simulink model "Sim6_03_lim_current_LCL"  (R2019b)
settings: Solver=ode1  StartTime=0.0  StopTime=1.5  FixedStep=Time_Step  MaxStep=1e-5  RelTol=1e-3
undefined symbols (not defined in the file): C_line, L_1, L_2, R_1, R_2, Theta0, Time_Step, Un, V0, VSC01_id0
libraries: powerlib x37, Control_Lib x7, simulink x5, powerlib_meascontrol x4
(part 2 of 2)

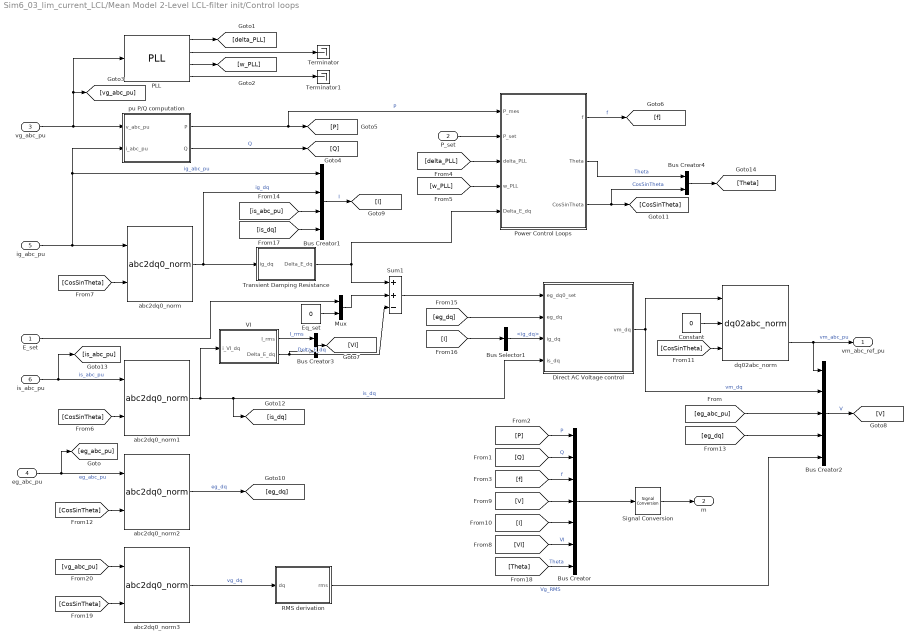
== system Sim6_03_lim_current_LCL/Mean Model 2-Level LCL-filter init/Control loops ==
  E_set : Inport
  P_set : Inport  Port=2
  vg_abc_pu : Inport  Port=3
  eg_abc_pu : Inport  Port=4
  ig_abc_pu : Inport  Port=5
  is_abc_pu : Inport  Port=6
  " pu P/Q computation" : Subsystem  DialogController=POWERSYS.PowerSysDialog
  Bus Creator : BusCreator  Inputs=7
  Bus Creator1 : BusCreator  Inputs=4
  Bus Creator2 : BusCreator  Inputs=5
  Bus Creator3 : BusCreator  Inputs=2
  Bus Creator4 : BusCreator  Inputs=2
  Bus Selector1 : BusSelector  OutputSignals=ig_dq
  Constant : Constant  Value=0
  Direct AC Voltage control : Subsystem
  Eq_set : Constant  Value=0
  Mux : Mux  Inputs=2
  PLL : Control_Lib/PLL  fb=fb  Tr_PLL=Tr_PLL  Theta0=Theta0
      settings: SourceProductName=VSC4SPS
  Power Control Loops : Subsystem
  RMS derivation : Subsystem
  Signal Conversion : SignalConversion  OverrideOpt=off
  Sum1 : Sum  Inputs=++-
  Terminator : Terminator
  Terminator1 : Terminator
  Transient Damping Resistance : Subsystem
  VI : Subsystem
  abc2dq0_norm{,1..3} (4 alike) : Control_Lib/abc2dq0_norm  referenceAxisMode=Reference axis at 90 degrees behind phase_a  baseUpdateGain=1/sqrt(3)
      settings: SourceProductName=VSC4SPS
  dq02abc_norm : Control_Lib/dq02abc_norm  referenceAxisMode=Reference axis at 90 degrees behind phase_a  baseUpdateGain=sqrt(3)
      settings: SourceProductName=VSC4SPS
  vm_abc_ref_pu : Outport  PortDimensions=3  VectorParamsAs1DForOutWhenUnconnected=off
  m : Outport  Port=2  VectorParamsAs1DForOutWhenUnconnected=off
  wires:
  [w_PLL] -> Power Control Loops/4(w_PLL)
  RMS derivation/1(rms) -> Bus Creator2/5  "Vg_RMS"
  abc2dq0_norm3/2 -> RMS derivation/1(dq)  "vg_dq"
  [vg_abc_pu] -> abc2dq0_norm3/1
  [CosSinTheta] -> abc2dq0_norm3/2
  [Theta] -> Bus Creator/7  "Theta"
  Bus Creator4/1 -> [Theta]
  Power Control Loops/2(Theta) -> Bus Creator4/1  "Theta"
  Power Control Loops/3(CosSinTheta) -> [CosSinTheta], Bus Creator4/2  "CosSinTheta"
  PLL/4 -> Terminator1/1
  PLL/2 -> Terminator/1
  Constant/1 -> dq02abc_norm/2
  PLL/3 -> [w_PLL]
  PLL/1 -> [delta_PLL]
  Sum1/1 -> Direct AC Voltage control/1(eg_dq0_set)
  [I] -> Bus Selector1/1
  Bus Selector1/1 -> Direct AC Voltage control/3(ig_dq)  "<ig_dq>"
  Bus Creator2/1 -> [V]  "V"
  [CosSinTheta] -> dq02abc_norm/3
  dq02abc_norm/2 -> vm_abc_ref_pu/1, Bus Creator2/1  "vm_abc_pu"
  Direct AC Voltage control/1(vm_dq) -> Bus Creator2/2, dq02abc_norm/1  "vm_dq"
  [eg_dq] -> Direct AC Voltage control/2(eg_dq)
  eg_abc_pu/1 -> [eg_abc_pu], abc2dq0_norm2/1  "eg_abc_pu"
  is_abc_pu/1 -> abc2dq0_norm1/1, [is_abc_pu]  "is_abc_pu"
  abc2dq0_norm2/2 -> [eg_dq]  "eg_dq"
  [CosSinTheta] -> abc2dq0_norm2/2
  abc2dq0_norm1/2 -> [is_dq], Direct AC Voltage control/4(is_dq), VI/1(i_VI_dq)  "is_dq"
  vg_abc_pu/1 -> PLL/1, [vg_abc_pu], " pu P/Q computation"/1(v_abc_pu)
  [CosSinTheta] -> abc2dq0_norm1/2
  [I] -> Bus Creator/5
  Bus Creator1/1 -> [I]  "I"
  Bus Creator/1 -> Signal Conversion/1
  [VI] -> Bus Creator/6  "VI"
  [V] -> Bus Creator/4
  Eq_set/1 -> Mux/2
  Mux/1 -> Sum1/2
  VI/1(I_rms) -> Bus Creator3/1  "I_rms"
  Transient Damping Resistance/1("Delta_E_dq ") -> Sum1/1, Power Control Loops/5(Delta_E_dq)
  VI/2(Delta_E_dq) -> Sum1/3, Bus Creator3/2  "Delta_E_dq"
  [CosSinTheta] -> abc2dq0_norm/2
  abc2dq0_norm/2 -> Transient Damping Resistance/1(ig_dq), Bus Creator1/2  "ig_dq"
  ig_abc_pu/1 -> " pu P/Q computation"/2(i_abc_pu), Bus Creator1/1, abc2dq0_norm/1  "ig_abc_pu"
  " pu P/Q computation"/1(P) -> [P], Power Control Loops/1(P_mes)  "P"
  Power Control Loops/1(f) -> [f]  "f"
  P_set/1 -> Power Control Loops/2(P_set)
  [delta_PLL] -> Power Control Loops/3(delta_PLL)
  " pu P/Q computation"/2(Q) -> [Q]  "Q"
  E_set/1 -> Mux/1
  [f] -> Bus Creator/3  "f"
  [Q] -> Bus Creator/2  "Q"
  [P] -> Bus Creator/1  "P"
  Signal Conversion/1 -> m/1
  Bus Creator3/1 -> [VI]
  [eg_abc_pu] -> Bus Creator2/3
  [eg_dq] -> Bus Creator2/4
  [is_abc_pu] -> Bus Creator1/3
  [is_dq] -> Bus Creator1/4

== system Sim6_03_lim_current_LCL/Mean Model 2-Level LCL-filter init/Output_Filter ==
  Filter capacitance : powerlib/Elements/Three-Phase Series RLC Branch  LConnTagsString=A|B|C  RConnTagsString=A|B|C  BranchType=C  Resistance=0  Inductance=C_line(1)  Capacitance=Cf_pu*Cb  Measurements=None
  Filter inductance : powerlib/Elements/Three-Phase Series RLC Branch  LConnTagsString=A|B|C  RConnTagsString=A|B|C  BranchType=RL  Resistance=Rf_pu*Zb  Inductance=Lf_pu*Lb  Capacitance=1e-6  Measurements=None
  Ground : powerlib/Elements/Ground  LConnTagsString=a
  A : PMIOPort  Side=Left
  a : PMIOPort  Port=2  Side=Right
  B : PMIOPort  Port=3  Side=Left
  b : PMIOPort  Port=4  Side=Right
  C : PMIOPort  Port=5  Side=Left
  c : PMIOPort  Port=6  Side=Right
  connections:
  Ground/LConn1 -- Filter capacitance/RConn1 -- Filter capacitance/RConn3 -- Filter capacitance/RConn2
  b/RConn1 -- Filter capacitance/LConn2 -- Filter inductance/RConn2
  Filter inductance/LConn1 -- A/RConn1
  Filter inductance/LConn3 -- C/RConn1
  Filter inductance/LConn2 -- B/RConn1
  c/RConn1 -- Filter capacitance/LConn3 -- Filter inductance/RConn3
  a/RConn1 -- Filter capacitance/LConn1 -- Filter inductance/RConn1

== system Sim6_03_lim_current_LCL/Infinite_Grid/InertialDqVoltageSource/NetworkLeadLagTimeConstants ==
  In1 : Inport
  Integrator3 : Integrator  InitialCondition=(P0/Sb)*(1-TN/TD)
  Sum1 : Sum
  Sum2 : Sum  Inputs=+-
  mp1 : Gain  Gain=TN/TD
  mp2 : Gain  Gain=1-TN/TD
  mp3 : Gain  Gain=1/TD
  Out1 : Outport  VectorParamsAs1DForOutWhenUnconnected=off
  wires:
  Sum2/1 -> mp3/1
  mp3/1 -> Integrator3/1
  Integrator3/1 -> Sum1/2, Sum2/2
  In1/1 -> mp1/1, mp2/1
  mp2/1 -> Sum2/1
  mp1/1 -> Sum1/1
  Sum1/1 -> Out1/1

== system Sim6_03_lim_current_LCL/Infinite_Grid/Source_For_OP/Subsystem3 ==
  switch : Inport
  Breaker : powerlib/Elements/Breaker  InitialState=0  SwitchingTimes="[1/60  5/60]"  External=on  BreakerResistance=0.001  SnubberResistance=1e6  SnubberCapacitance=inf  Measurements=None  MoreParameters=on  NoBreakLoop=off
  Breaker1 : powerlib/Elements/Breaker  InitialState=0  SwitchingTimes="[1/60  5/60]"  External=on  BreakerResistance=0.001  SnubberResistance=1e6  SnubberCapacitance=inf  Measurements=None  MoreParameters=on  NoBreakLoop=off
  Breaker2 : powerlib/Elements/Breaker  InitialState=0  SwitchingTimes="[1/60  5/60]"  External=on  BreakerResistance=0.001  SnubberResistance=1e6  SnubberCapacitance=inf  Measurements=None  MoreParameters=on  NoBreakLoop=off
  Breaker3 : powerlib/Elements/Breaker  InitialState=1  SwitchingTimes="[1/60  5/60]"  External=on  BreakerResistance=0.001  SnubberResistance=1e6  SnubberCapacitance=inf  Measurements=None  MoreParameters=on  NoBreakLoop=off
  Breaker4 : powerlib/Elements/Breaker  InitialState=1  SwitchingTimes="[1/60  5/60]"  External=on  BreakerResistance=0.001  SnubberResistance=1e6  SnubberCapacitance=inf  Measurements=None  MoreParameters=on  NoBreakLoop=off
  Breaker5 : powerlib/Elements/Breaker  InitialState=1  SwitchingTimes="[1/60  5/60]"  External=on  BreakerResistance=0.001  SnubberResistance=1e6  SnubberCapacitance=inf  Measurements=None  MoreParameters=on  NoBreakLoop=off
  Logical Operator : Logic  Operator=NOT  AllPortsSameDT=off  OutDataTypeStr=boolean
  A : PMIOPort  Side=Left
  B : PMIOPort  Port=2  Side=Left
  C : PMIOPort  Port=3  Side=Left
  Ainit : PMIOPort  Port=4  Side=Left
  Binit : PMIOPort  Port=5  Side=Left
  Cinit : PMIOPort  Port=6  Side=Left
  a : PMIOPort  Port=7  Side=Right
  b : PMIOPort  Port=8  Side=Right
  c : PMIOPort  Port=9  Side=Right
  wires:
  Logical Operator/1 -> Breaker3/1, Breaker4/1, Breaker5/1
  switch/1 -> Logical Operator/1, Breaker/1, Breaker1/1, Breaker2/1
  connections:
  Breaker4/RConn1 -- Breaker1/RConn1 -- b/RConn1
  a/RConn1 -- Breaker3/RConn1 -- Breaker/RConn1
  Breaker1/LConn1 -- B/RConn1
  Breaker3/LConn1 -- Ainit/RConn1
  Breaker2/LConn1 -- C/RConn1
  Breaker4/LConn1 -- Binit/RConn1
  Breaker2/RConn1 -- Breaker5/RConn1 -- c/RConn1
  Breaker5/LConn1 -- Cinit/RConn1
  Breaker/LConn1 -- A/RConn1

== system Sim6_03_lim_current_LCL/Mean Model 2-Level LCL-filter init/Bridge_Model/Detailed ==
  Urref : Inport
  Bus Selector : BusSelector  OutputSignals=carrier
  PWM Generator (2-Level) : powerlib_meascontrol/Pulse & Signal Generators/PWM Generator (2-Level)  ModulatorType=Three-phase bridge (6 pulses)  ModulatorMode=Unsynchronized  Fc=fpwm  Pc=90  nF=27  MinMax="[ -1  1 ]"  SamplingTechnique=Natural  ModulatingSignals=off  m=0.8  Freq=60  Phase=0  Ts=Time_Step  ShowCarrierOutport=on
  Scope : Scope
  Scope1 : Scope
  Universal Bridge1 : powerlib/Power Electronics/Universal Bridge  Arms=3  SnubberResistance=1e5  SnubberCapacitance=inf  Device=IGBT / Diodes  Ron=1e-3  Lon=0  ForwardVoltages="[  0  0  ]"  ForwardVoltage=0  GTOparameters=[ 10e-6 , 20e-6 ]  IGBTparameters=[ 1e-6 , 2e-6 ]  Measurements=None  Measurements_2=None  converterType=Rectifier
  + : PMIOPort  Side=Right
  A : PMIOPort  Port=2  Side=Left
  B : PMIOPort  Port=3  Side=Left
  - : PMIOPort  Port=4  Side=Right
  C : PMIOPort  Port=5  Side=Left
  wires:
  PWM Generator (2-Level)/1 -> Universal Bridge1/1, Scope1/1
  Urref/1 -> PWM Generator (2-Level)/1
  PWM Generator (2-Level)/2 -> Bus Selector/1
  Bus Selector/1 -> Scope/1  "<carrier>"
  connections:
  Universal Bridge1/LConn3 -- C/RConn1
  Universal Bridge1/LConn1 -- A/RConn1
  Universal Bridge1/LConn2 -- B/RConn1
  Universal Bridge1/RConn2 -- -/RConn1
  Universal Bridge1/RConn1 -- +/RConn1

== system Sim6_03_lim_current_LCL/Mean Model 2-Level LCL-filter init/Control loops/ pu P//Q computation ==
  v_abc_pu : Inport  PortDimensions=3
  i_abc_pu : Inport  Port=2  PortDimensions=3
  Demux : Demux  Outputs=3
      settings: DisplayOption=none
  Mux : Mux  Inputs=3
  Product1 : Product  InputSameDT=on  SaturateOnIntegerOverflow=on  OutDataTypeStr=Inherit: Same as first input
  Product3 : Product  InputSameDT=on  SaturateOnIntegerOverflow=on  OutDataTypeStr=Inherit: Same as first input
  Sum : Sum  Inputs=+-  InputSameDT=on  SaturateOnIntegerOverflow=on  OutDataTypeStr=Inherit: Same as first input
  Sum1 : Sum  Inputs=1  InputSameDT=on  SaturateOnIntegerOverflow=on  OutDataTypeStr=Inherit: Same as first input
  Sum4 : Sum  Inputs=1  InputSameDT=on  SaturateOnIntegerOverflow=on  OutDataTypeStr=Inherit: Same as first input
  Sum5 : Sum  Inputs=+-  InputSameDT=on  SaturateOnIntegerOverflow=on  OutDataTypeStr=Inherit: Same as first input
  Sum6 : Sum  Inputs=+-  InputSameDT=on  SaturateOnIntegerOverflow=on  OutDataTypeStr=Inherit: Same as first input
  pu->V : Gain  Gain=1/sqrt(3)  SaturateOnIntegerOverflow=on  OutDataTypeStr=Inherit: Same as input  ParamDataTypeStr=Inherit: Same as input
  pu->V1 : Gain  Gain=1/3  SaturateOnIntegerOverflow=on  OutDataTypeStr=Inherit: Same as input  ParamDataTypeStr=Inherit: Same as input
  pu->V2 : Gain  Gain=1/3  SaturateOnIntegerOverflow=on  OutDataTypeStr=Inherit: Same as input  ParamDataTypeStr=Inherit: Same as input
  P : Outport  VectorParamsAs1DForOutWhenUnconnected=off
  Q : Outport  Port=2  VectorParamsAs1DForOutWhenUnconnected=off
  wires:
  pu->V2/1 -> Q/1
  pu->V1/1 -> P/1
  Sum1/1 -> pu->V/1
  Product3/1 -> Sum1/1
  Product1/1 -> Sum4/1
  v_abc_pu/1 -> Product1/1, Demux/1
  i_abc_pu/1 -> Product1/2, Product3/2
  Sum4/1 -> pu->V1/1
  Demux/1 -> Sum/1, Sum6/2
  Demux/2 -> Sum/2, Sum5/1
  Demux/3 -> Sum5/2, Sum6/1
  Sum/1 -> Mux/3
  Sum5/1 -> Mux/1
  Sum6/1 -> Mux/2
  Mux/1 -> Product3/1
  pu->V/1 -> pu->V2/1  "Q"

== system Sim6_03_lim_current_LCL/Mean Model 2-Level LCL-filter init/Control loops/Direct AC Voltage control ==
  note: direct AC voltage control
  eg_dq0_set : Inport
  eg_dq : Inport  Port=2
  ig_dq : Inport  Port=3
  is_dq : Inport  Port=4
  Current Limitation : Subsystem
  Gain : Gain  Gain=RLCL_D
  Gain2 : Gain  Gain=[Rf_pu -Lf_pu;Lf_pu Rf_pu]  Multiplication=Matrix(K*u)
  Second-Order Filter : powerlib_meascontrol/Filters/Second-Order Filter  FilterType=Highpass  Fo=f_damping  Zeta=1  Ts=0  Initialize=on  Vac_Init="[0,  0,  60; 0, 0, 60]"  Vdc_Init=[0, 0]  PlotResponse=off  FreqRange=[0, 500, 1]
      settings: SourceProductBaseCode=PS
  Second-Order Filter1 : powerlib_meascontrol/Filters/Second-Order Filter  FilterType=Lowpass  Fo=f_damping  Zeta=1  Ts=0  Initialize=on  Vac_Init="[0,  0,  60; 0 0 60]"  Vdc_Init=[Is0_d; Is0_q]  PlotResponse=off  FreqRange=[0, 500, 1]
      settings: SourceProductBaseCode=PS
  Second-Order Filter2 : powerlib_meascontrol/Filters/Second-Order Filter  FilterType=Lowpass  Fo=1000  Zeta=1  Ts=0  Initialize=on  Vac_Init="[0,  0,  60; 0, 0, 60]"  Vdc_Init=[0, 0]  PlotResponse=off  FreqRange=[0, 500, 1]
      settings: SourceProductBaseCode=PS
  Sum : Sum  Inputs=|++
  Sum1 : Sum  Inputs=|+-
  Sum2 : Sum  Inputs=-+|
  vm_dq : Outport  VectorParamsAs1DForOutWhenUnconnected=off
  wires:
  ig_dq/1 -> Sum1/2
  eg_dq/1 -> Current Limitation/3(Eg_dq)
  is_dq/1 -> Second-Order Filter1/1, Current Limitation/2(Is_dq), Sum1/1
  eg_dq0_set/1 -> Sum/2
  Sum/1 -> Sum2/2
  Sum1/1 -> Second-Order Filter/1
  Second-Order Filter/1 -> Second-Order Filter2/1
  Gain/1 -> Sum2/1
  Sum2/1 -> Current Limitation/1(Vm_dq*)
  Gain2/1 -> Sum/1
  Second-Order Filter1/1 -> Gain2/1
  Second-Order Filter2/1 -> Gain/1
  Current Limitation/1(Vm_dq_sat) -> vm_dq/1

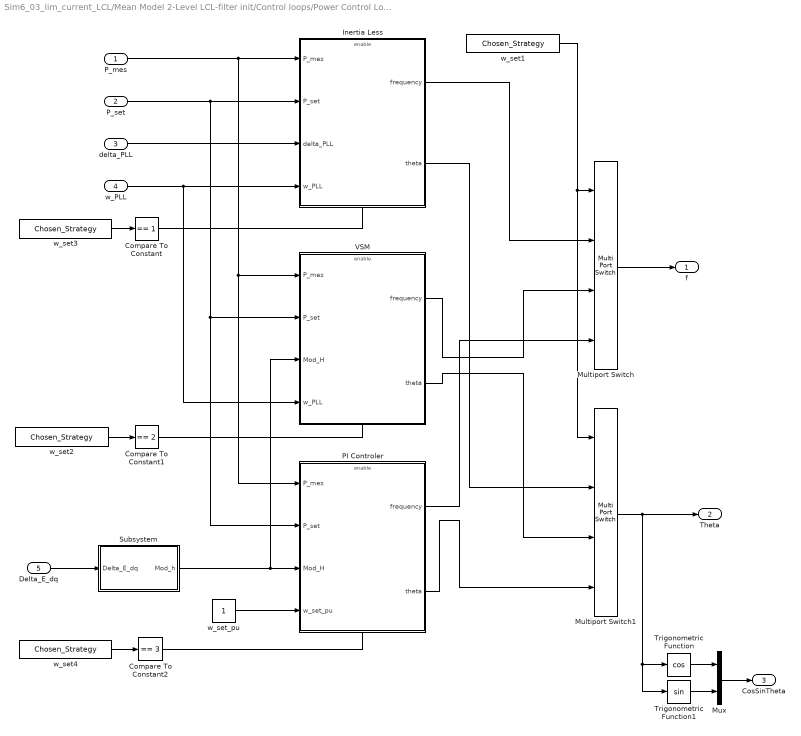
== system Sim6_03_lim_current_LCL/Mean Model 2-Level LCL-filter init/Control loops/Power Control Loops ==
  P_mes : Inport
  P_set : Inport  Port=2
  delta_PLL : Inport  Port=3
  w_PLL : Inport  Port=4
  Delta_E_dq : Inport  Port=5
  Compare To Constant : simulink/Logic and Bit Operations/Compare To Constant  relop===  const=1  OutDataTypeStr=boolean
  Compare To Constant1 : simulink/Logic and Bit Operations/Compare To Constant  relop===  const=2  OutDataTypeStr=boolean
  Compare To Constant2 : simulink/Logic and Bit Operations/Compare To Constant  relop===  const=3  OutDataTypeStr=boolean
  Inertia Less : Subsystem
  Multiport Switch : MultiPortSwitch
  Multiport Switch1 : MultiPortSwitch
  Mux : Mux  Inputs=[1 1]
  PI Controler : Subsystem
  Subsystem : Subsystem
  Trigonometric Function : Trigonometry  Operator=cos
  Trigonometric Function1 : Trigonometry
  VSM : Subsystem
  w_set{1..4} (4 alike) : Constant  Value=Chosen_Strategy
  w_set_pu : Constant
  f : Outport  PortDimensions=1  VectorParamsAs1DForOutWhenUnconnected=off
  Theta : Outport  Port=2  VectorParamsAs1DForOutWhenUnconnected=off
  CosSinTheta : Outport  Port=3  PortDimensions=2  VectorParamsAs1DForOutWhenUnconnected=off
  wires:
  P_mes/1 -> PI Controler/1(P_mes), VSM/1(P_mes), Inertia Less/1(P_mes)
  P_set/1 -> PI Controler/2(P_set), VSM/2(P_set), Inertia Less/2(P_set)
  delta_PLL/1 -> Inertia Less/3(delta_PLL)
  w_PLL/1 -> VSM/4(w_PLL), Inertia Less/4(w_PLL)
  w_set_pu/1 -> PI Controler/4(w_set_pu)
  PI Controler/2(theta) -> Multiport Switch1/4
  PI Controler/1(frequency) -> Multiport Switch/4
  VSM/1(frequency) -> Multiport Switch/3
  w_set1/1 -> Multiport Switch1/1, Multiport Switch/1
  VSM/2(theta) -> Multiport Switch1/3
  Inertia Less/2(theta) -> Multiport Switch1/2
  Multiport Switch/1 -> f/1
  Inertia Less/1(frequency) -> Multiport Switch/2
  w_set3/1 -> Compare To Constant/1
  w_set2/1 -> Compare To Constant1/1
  w_set4/1 -> Compare To Constant2/1
  Compare To Constant/1 -> Inertia Less/Enable
  Compare To Constant1/1 -> VSM/Enable
  Compare To Constant2/1 -> PI Controler/Enable
  Trigonometric Function/1 -> Mux/1
  Mux/1 -> CosSinTheta/1
  Trigonometric Function1/1 -> Mux/2
  Multiport Switch1/1 -> Theta/1, Trigonometric Function/1, Trigonometric Function1/1
  Delta_E_dq/1 -> Subsystem/1(Delta_E_dq)
  Subsystem/1(Mod_h) -> VSM/3(Mod_H), PI Controler/3(Mod_H)

== system Sim6_03_lim_current_LCL/Mean Model 2-Level LCL-filter init/Control loops/RMS derivation ==
  dq : Inport
  Demux : Demux  Outputs=2
  Sqrt : Sqrt  SaturateOnIntegerOverflow=on
  Square : Math  Operator=square  SaturateOnIntegerOverflow=on
  Square1 : Math  Operator=square  SaturateOnIntegerOverflow=on
  Sum : Sum
  rms : Outport
  wires:
  Square1/1 -> Sum/2
  Sum/1 -> Sqrt/1
  Sqrt/1 -> rms/1
  Demux/1 -> Square/1
  Square/1 -> Sum/1
  Demux/2 -> Square1/1
  dq/1 -> Demux/1

== system Sim6_03_lim_current_LCL/Mean Model 2-Level LCL-filter init/Control loops/Transient Damping Resistance ==
  ig_dq : Inport
  Filter w_LF : Subsystem
      mask Display: disp('\omega_{LF} / (s + \omega_{LF})','texmode','on')
  Sum5 : Sum  Inputs=|+-
  nq1 : Gain  Gain=Rv
  "Delta_E_dq " : Outport  VectorParamsAs1DForOutWhenUnconnected=off
  wires:
  nq1/1 -> Filter w_LF/1(e), Sum5/2
  Filter w_LF/1(s) -> Sum5/1
  Sum5/1 -> "Delta_E_dq "/1
  ig_dq/1 -> nq1/1

== system Sim6_03_lim_current_LCL/Mean Model 2-Level LCL-filter init/Control loops/VI ==
  note: VI triggering and threshold computation
  note: VI
  i_VI_dq : Inport
  Demux1 : Demux  Outputs=2
      settings: DisplayOption=none
  Gain5 : Gain  Gain=DX_DR
  Gain6 : Gain  Gain=Kp_Rvi_pu
  Gain9 : Gain  Gain=DX_DR
  I_thresh : Constant
  Mux2 : Mux  Inputs=2
  Saturation : Saturate  UpperLimit=inf  LowerLimit=0
  Sum1 : Sum  Inputs=-+|
  Sum7 : Sum  Inputs=|+-
  Sum8 : Sum  Inputs=++|
  dq to phasor : Subsystem
  product{,1..3} (4 alike) : Product  InputSameDT=on  RndMeth=Zero  SaturateOnIntegerOverflow=on  OutDataTypeStr=Inherit: Same as first input
  I_rms : Outport  VectorParamsAs1DForOutWhenUnconnected=off
  Delta_E_dq : Outport  Port=2  VectorParamsAs1DForOutWhenUnconnected=off
  wires:
  Sum1/1 -> Saturation/1
  dq to phasor/1(rms) -> I_rms/1, Sum1/2  "I_rms"
  Saturation/1 -> Gain6/1
  I_thresh/1 -> Sum1/1
  Mux2/1 -> Delta_E_dq/1
  Gain6/1 -> product3/2, product/1, product1/2, product2/2
  product3/1 -> Gain5/1
  product/1 -> Gain9/1
  Demux1/1 -> product1/1, product/2  "igd"
  Demux1/2 -> product2/1, product3/1  "igq"
  product1/1 -> Sum7/1
  Gain5/1 -> Sum7/2
  Gain9/1 -> Sum8/1
  product2/1 -> Sum8/2
  Sum7/1 -> Mux2/1
  Sum8/1 -> Mux2/2
  i_VI_dq/1 -> dq to phasor/1(dq_mes), Demux1/1

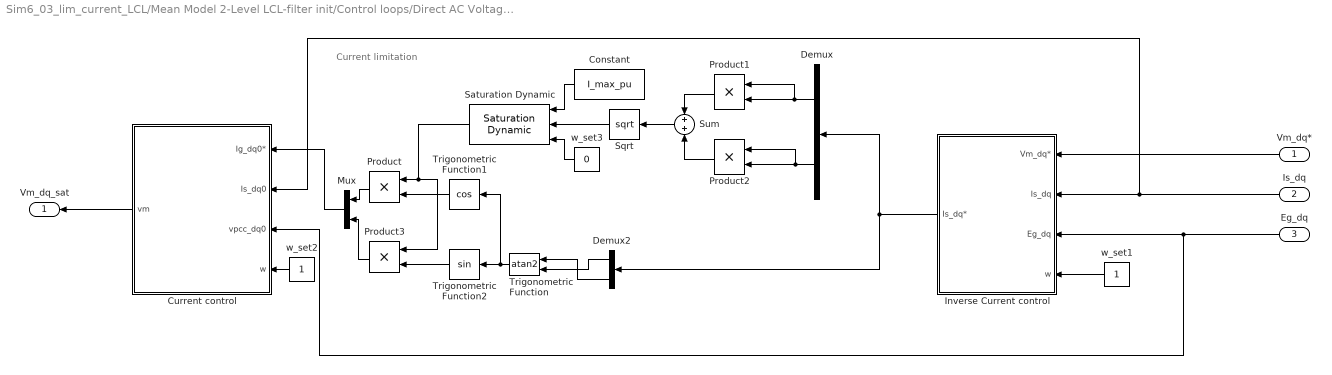
== system Sim6_03_lim_current_LCL/Mean Model 2-Level LCL-filter init/Control loops/Direct AC Voltage control/Current Limitation ==
  note: Current limitation
  Vm_dq* : Inport
  Is_dq : Inport  Port=2
  Eg_dq : Inport  Port=3
  Constant : Constant  Value=I_max_pu
  Current control : Subsystem
  Demux : Demux  Outputs=2
  Demux2 : Demux  Outputs=2
  Inverse Current control : Subsystem
  Mux : Mux  Inputs=2
  Product{,1..3} (4 alike) : Product
  Saturation Dynamic : simulink/Discontinuities/Saturation Dynamic  OutMin=[]  OutMax=[]  OutDataTypeStr=Inherit: Same as second input  OutDataType=fixdt(1, 16)  OutScaling=2^-10  DoSatur=off
  Sqrt : Sqrt  SaturateOnIntegerOverflow=on
  Sum : Sum
  Trigonometric Function : Trigonometry  Operator=atan2  NumberOfIterations=5  OutputSignalType=real
  Trigonometric Function1 : Trigonometry  Operator=cos
  Trigonometric Function2 : Trigonometry
  w_set1 : Constant
  w_set2 : Constant
  w_set3 : Constant  Value=0
  Vm_dq_sat : Outport  VectorParamsAs1DForOutWhenUnconnected=off
  wires:
  w_set3/1 -> Saturation Dynamic/3
  Constant/1 -> Saturation Dynamic/1
  Mux/1 -> Current control/1(Ig_dq0*)
  Product/1 -> Mux/1
  Demux/1 -> Product1/1, Product1/2
  Demux/2 -> Product2/1, Product2/2
  Trigonometric Function2/1 -> Product3/2
  Product2/1 -> Sum/2
  Trigonometric Function1/1 -> Product/2
  Demux2/1 -> Trigonometric Function/2
  Trigonometric Function/1 -> Trigonometric Function2/1, Trigonometric Function1/1
  Saturation Dynamic/1 -> Product/1, Product3/1
  Product1/1 -> Sum/1
  Sqrt/1 -> Saturation Dynamic/2
  Demux2/2 -> Trigonometric Function/1
  Inverse Current control/1(Is_dq*) -> Demux2/1, Demux/1
  Sum/1 -> Sqrt/1
  Product3/1 -> Mux/2
  Is_dq/1 -> Inverse Current control/2(Is_dq), Current control/2(Is_dq0)
  w_set1/1 -> Inverse Current control/4(w)
  w_set2/1 -> Current control/4(w)
  Eg_dq/1 -> Current control/3(vpcc_dq0), Inverse Current control/3(Eg_dq)
  Vm_dq*/1 -> Inverse Current control/1(Vm_dq*)
  Current control/1(vm) -> Vm_dq_sat/1

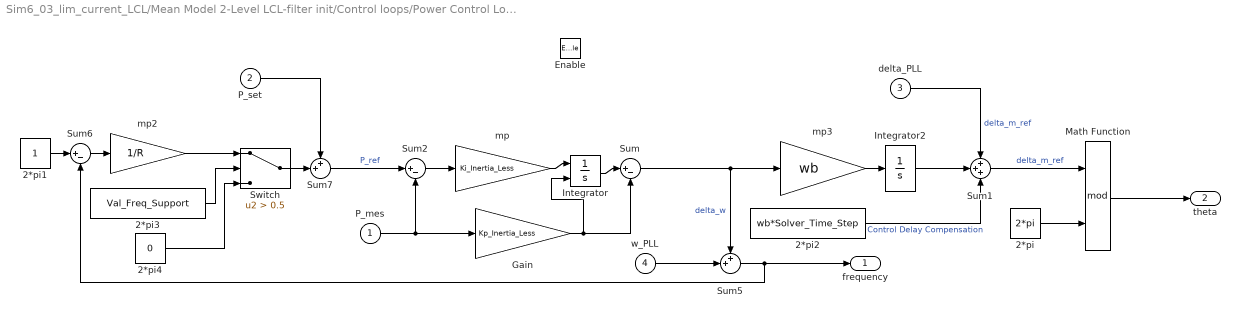
== system Sim6_03_lim_current_LCL/Mean Model 2-Level LCL-filter init/Control loops/Power Control Loops/Inertia Less ==
  P_mes : Inport
  P_set : Inport  Port=2
  delta_PLL : Inport  Port=3
  w_PLL : Inport  Port=4
  Enable : EnablePort
  2*pi : Constant  Value=2*pi
  2*pi1 : Constant
  2*pi2 : Constant  Value=wb*Solver_Time_Step
  2*pi3 : Constant  Value=Val_Freq_Support
  2*pi4 : Constant  Value=0
  Gain : Gain  Gain=Kp_Inertia_Less
  Integrator : Integrator  InitialConditionSource=external
  Integrator2 : Integrator  InitialCondition=(Theta_m0)*pi/180-Theta0*pi/180
  Math Function : Math  Operator=mod  SignedPower=on  SaturateOnIntegerOverflow=on
  Sum : Sum  Inputs=|+-
  Sum1 : Sum  Inputs=+++
  Sum2 : Sum  Inputs=|+-
  Sum5 : Sum  Inputs=++|
  Sum6 : Sum  Inputs=|+-
  Sum7 : Sum  Inputs=++|
  Switch : Switch  Criteria=u2 > Threshold  Threshold=0.5
  mp : Gain  Gain=Ki_Inertia_Less
  mp2 : Gain  Gain=1/R
  mp3 : Gain  Gain=wb
  frequency : Outport  VectorParamsAs1DForOutWhenUnconnected=off
  theta : Outport  Port=2  VectorParamsAs1DForOutWhenUnconnected=off
  wires:
  Sum2/1 -> mp/1
  Sum1/1 -> Math Function/1  "delta_m_ref"
  2*pi/1 -> Math Function/2
  2*pi1/1 -> Sum6/1
  Sum6/1 -> mp2/1
  P_set/1 -> Sum7/1
  Sum7/1 -> Sum2/1  "P_ref"
  P_mes/1 -> Gain/1, Sum2/2
  Switch/1 -> Sum7/2
  Math Function/1 -> theta/1
  Sum/1 -> mp3/1, Sum5/1  "delta_w"
  mp3/1 -> Integrator2/1
  mp/1 -> Integrator/1
  delta_PLL/1 -> Sum1/1  "delta_m_ref"
  w_PLL/1 -> Sum5/2
  Sum5/1 -> frequency/1, Sum6/2
  2*pi2/1 -> Sum1/3  "Control Delay Compensation"
  Integrator2/1 -> Sum1/2
  mp2/1 -> Switch/1
  2*pi3/1 -> Switch/2
  2*pi4/1 -> Switch/3
  Integrator/1 -> Sum/1
  Gain/1 -> Integrator/2, Sum/2

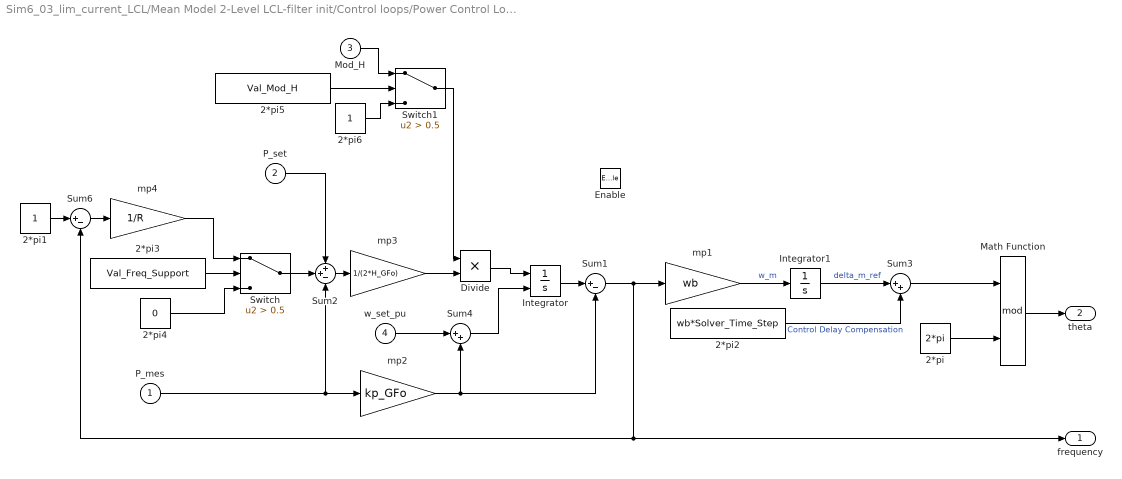
== system Sim6_03_lim_current_LCL/Mean Model 2-Level LCL-filter init/Control loops/Power Control Loops/PI Controler ==
  P_mes : Inport
  P_set : Inport  Port=2
  Mod_H : Inport  Port=3
  w_set_pu : Inport  Port=4
  Enable : EnablePort
  2*pi : Constant  Value=2*pi
  2*pi1 : Constant
  2*pi2 : Constant  Value=wb*Solver_Time_Step
  2*pi3 : Constant  Value=Val_Freq_Support
  2*pi4 : Constant  Value=0
  2*pi5 : Constant  Value=Val_Mod_H
  2*pi6 : Constant
  Divide : Product  Inputs=**
  Integrator : Integrator  InitialConditionSource=external
  Integrator1 : Integrator  InitialCondition=(Theta_m0)*pi/180
  Math Function : Math  Operator=mod  SignedPower=on  SaturateOnIntegerOverflow=on
  Sum1 : Sum  Inputs=|+-
  Sum2 : Sum  Inputs=++-
  Sum3 : Sum  Inputs=|++
  Sum4 : Sum  Inputs=|++
  Sum6 : Sum  Inputs=|+-
  Switch : Switch  Criteria=u2 > Threshold  Threshold=0.5
  Switch1 : Switch  Criteria=u2 > Threshold  Threshold=0.5
  mp1 : Gain  Gain=wb
  mp2 : Gain  Gain=kp_GFo
  mp3 : Gain  Gain=1/(2*H_GFo)
  mp4 : Gain  Gain=1/R
  frequency : Outport  VectorParamsAs1DForOutWhenUnconnected=off
  theta : Outport  Port=2  VectorParamsAs1DForOutWhenUnconnected=off
  wires:
  Sum2/1 -> mp3/1
  Integrator1/1 -> Sum3/1  "delta_m_ref"
  Math Function/1 -> theta/1
  2*pi/1 -> Math Function/2
  w_set_pu/1 -> Sum4/1
  P_set/1 -> Sum2/1
  Integrator/1 -> Sum1/1
  Sum1/1 -> mp1/1, frequency/1, Sum6/2
  mp1/1 -> Integrator1/1  "w_m"
  Sum3/1 -> Math Function/1
  2*pi2/1 -> Sum3/2  "Control Delay Compensation"
  P_mes/1 -> Sum2/3, mp2/1
  mp2/1 -> Sum1/2, Sum4/2
  mp3/1 -> Divide/2
  Sum4/1 -> Integrator/2
  mp4/1 -> Switch/1
  2*pi1/1 -> Sum6/1
  2*pi3/1 -> Switch/2
  Sum6/1 -> mp4/1
  2*pi4/1 -> Switch/3
  Switch/1 -> Sum2/2
  2*pi5/1 -> Switch1/2
  2*pi6/1 -> Switch1/3
  Mod_H/1 -> Switch1/1
  Divide/1 -> Integrator/1
  Switch1/1 -> Divide/1

== system Sim6_03_lim_current_LCL/Mean Model 2-Level LCL-filter init/Control loops/Power Control Loops/Subsystem ==
  Delta_E_dq : Inport
  Constant : Constant
  Constant1 : Constant  Value=2
  Delay : Delay  DelayLength=1  InitialCondition=1
  Demux : Demux  Outputs=2
  Pow : Math  Operator=pow  SignedPower=on  RndMeth=Zero  SaturateOnIntegerOverflow=on
  Square : Math  Operator=square  SignedPower=on  RndMeth=Zero  SaturateOnIntegerOverflow=on
  Square1 : Math  Operator=square  SignedPower=on  RndMeth=Zero  SaturateOnIntegerOverflow=on
  Sum : Sum  Inputs=|+-
  Sum5 : Sum
  Mod_h : Outport  VectorParamsAs1DForOutWhenUnconnected=off
  wires:
  Delta_E_dq/1 -> Delay/1
  Square/1 -> Sum5/1
  Pow/1 -> Mod_h/1
  Constant1/1 -> Pow/2
  Demux/2 -> Square1/1
  Constant/1 -> Sum/1
  Sum5/1 -> Pow/1
  Square1/1 -> Sum5/2
  Demux/1 -> Sum/2
  Sum/1 -> Square/1
  Delay/1 -> Demux/1

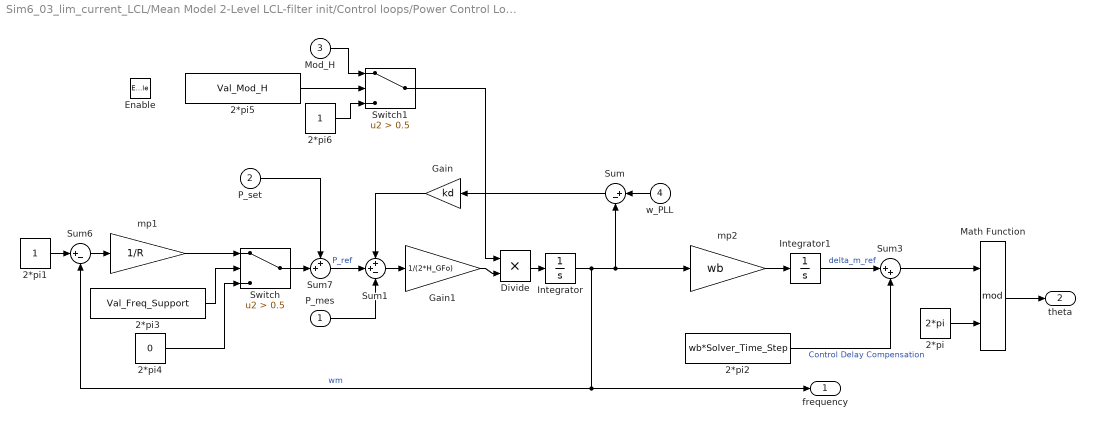
== system Sim6_03_lim_current_LCL/Mean Model 2-Level LCL-filter init/Control loops/Power Control Loops/VSM ==
  P_mes : Inport
  P_set : Inport  Port=2
  Mod_H : Inport  Port=3
  w_PLL : Inport  Port=4
  Enable : EnablePort
  2*pi : Constant  Value=2*pi
  2*pi1 : Constant
  2*pi2 : Constant  Value=wb*Solver_Time_Step
  2*pi3 : Constant  Value=Val_Freq_Support
  2*pi4 : Constant  Value=0
  2*pi5 : Constant  Value=Val_Mod_H
  2*pi6 : Constant
  Divide : Product  Inputs=**
  Gain : Gain  Gain=kd
  Gain1 : Gain  Gain=1/(2*H_GFo)
  Integrator : Integrator  InitialCondition=1
  Integrator1 : Integrator  InitialCondition=Theta_m0*pi/180
  Math Function : Math  Operator=mod  SignedPower=on  SaturateOnIntegerOverflow=on
  Sum : Sum  Inputs=|+-
  Sum1 : Sum  Inputs=++-
  Sum3 : Sum  Inputs=|++
  Sum6 : Sum  Inputs=|+-
  Sum7 : Sum  Inputs=++|
  Switch : Switch  Criteria=u2 > Threshold  Threshold=0.5
  Switch1 : Switch  Criteria=u2 > Threshold  Threshold=0.5
  mp1 : Gain  Gain=1/R
  mp2 : Gain  Gain=wb
  frequency : Outport  VectorParamsAs1DForOutWhenUnconnected=off
  theta : Outport  Port=2  VectorParamsAs1DForOutWhenUnconnected=off
  wires:
  2*pi/1 -> Math Function/2
  Math Function/1 -> theta/1
  Integrator1/1 -> Sum3/1  "delta_m_ref"
  Integrator/1 -> Sum/2, mp2/1, frequency/1, Sum6/2  "wm"
  P_mes/1 -> Sum1/3
  mp2/1 -> Integrator1/1
  2*pi2/1 -> Sum3/2  "Control Delay Compensation"
  Sum3/1 -> Math Function/1
  Switch/1 -> Sum7/2
  P_set/1 -> Sum7/1
  Sum6/1 -> mp1/1
  2*pi1/1 -> Sum6/1
  mp1/1 -> Switch/1
  2*pi3/1 -> Switch/2
  2*pi4/1 -> Switch/3
  w_PLL/1 -> Sum/1
  Sum/1 -> Gain/1
  Gain/1 -> Sum1/1
  Sum1/1 -> Gain1/1
  Sum7/1 -> Sum1/2  "P_ref"
  2*pi5/1 -> Switch1/2
  2*pi6/1 -> Switch1/3
  Mod_H/1 -> Switch1/1
  Divide/1 -> Integrator/1
  Gain1/1 -> Divide/2
  Switch1/1 -> Divide/1

== system Sim6_03_lim_current_LCL/Mean Model 2-Level LCL-filter init/Control loops/Transient Damping Resistance/Filter w_LF ==
  e : Inport
  1/T_LP : Gain  Gain=W_TVR  SaturateOnIntegerOverflow=on  OutDataTypeStr=Inherit: Same as input  ParamDataTypeStr=Inherit: Same as input
  Integrator : Integrator  InitialConditionSource=external  InitialCondition=[VSC01_id0*0.04]
  Sum1 : Sum  Inputs=|+-  InputSameDT=on  SaturateOnIntegerOverflow=on  OutDataTypeStr=Inherit: Same as first input
  s : Outport  VectorParamsAs1DForOutWhenUnconnected=off
  wires:
  e/1 -> Sum1/1, Integrator/2
  Integrator/1 -> s/1, Sum1/2
  1/T_LP/1 -> Integrator/1
  Sum1/1 -> 1/T_LP/1

== system Sim6_03_lim_current_LCL/Mean Model 2-Level LCL-filter init/Control loops/VI/dq to phasor ==
  dq_mes : Inport
  Demux : Demux  Outputs=2
      settings: DisplayOption=none
  Sqrt : Sqrt  SaturateOnIntegerOverflow=on
  Sum4 : Sum  Inputs=|++  InputSameDT=on  SaturateOnIntegerOverflow=on  OutDataTypeStr=Inherit: Same as first input
  Vrdird : Product  InputSameDT=on  RndMeth=Zero  SaturateOnIntegerOverflow=on  OutDataTypeStr=Inherit: Same as first input
  Vrqirq : Product  InputSameDT=on  RndMeth=Zero  SaturateOnIntegerOverflow=on  OutDataTypeStr=Inherit: Same as first input
  rms : Outport  VectorParamsAs1DForOutWhenUnconnected=off
  wires:
  Sum4/1 -> Sqrt/1
  Vrqirq/1 -> Sum4/2
  Vrdird/1 -> Sum4/1
  Demux/2 -> Vrqirq/2, Vrqirq/1
  Demux/1 -> Vrdird/2, Vrdird/1
  dq_mes/1 -> Demux/1
  Sqrt/1 -> rms/1

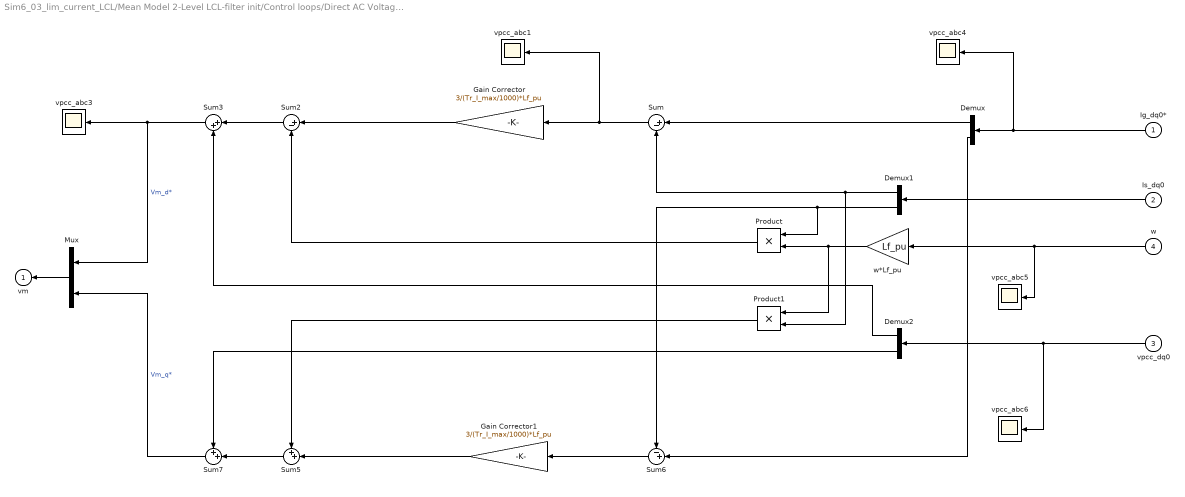
== system Sim6_03_lim_current_LCL/Mean Model 2-Level LCL-filter init/Control loops/Direct AC Voltage control/Current Limitation/Current control ==
  Ig_dq0* : Inport
  Is_dq0 : Inport  Port=2
  vpcc_dq0 : Inport  Port=3
  w : Inport  Port=4
  Demux : Demux  Outputs=2
  Demux1 : Demux  Outputs=2
  Demux2 : Demux  Outputs=2
  Gain Corrector : Gain  Gain=3/(Tr_I_max/1000)*Lf_pu
  Gain Corrector1 : Gain  Gain=3/(Tr_I_max/1000)*Lf_pu
  Mux : Mux  Inputs=2
  Product : Product  RndMeth=Zero
  Product1 : Product  RndMeth=Zero
  Sum : Sum  Inputs=|+-
  Sum2 : Sum  Inputs=|+-
  Sum3 : Sum  Inputs=|++
  Sum5 : Sum  Inputs=++|
  Sum6 : Sum  Inputs=-+|
  Sum7 : Sum  Inputs=++|
  vpcc_abc{1,3..6} (5 alike) : Scope
  w*Lf_pu : Gain  Gain=Lf_pu
  vm : Outport  InitialOutput=0  VectorParamsAs1DForOutWhenUnconnected=off
  wires:
  Demux2/2 -> Sum7/1
  Demux2/1 -> Sum3/2
  w/1 -> vpcc_abc5/1, w*Lf_pu/1
  Sum/1 -> vpcc_abc1/1, Gain Corrector/1
  Sum7/1 -> Mux/2  "Vm_q*"
  Sum3/1 -> Mux/1, vpcc_abc3/1  "Vm_d*"
  Sum5/1 -> Sum7/2
  Product1/1 -> Sum5/1
  Gain Corrector1/1 -> Sum5/2
  Demux/2 -> Sum6/2
  Sum2/1 -> Sum3/1
  Product/1 -> Sum2/2
  Demux1/2 -> Sum6/1, Product/1
  w*Lf_pu/1 -> Product/2, Product1/1
  Gain Corrector/1 -> Sum2/1
  Demux1/1 -> Sum/2, Product1/2
  Demux/1 -> Sum/1
  Is_dq0/1 -> Demux1/1
  vpcc_dq0/1 -> Demux2/1, vpcc_abc6/1
  Sum6/1 -> Gain Corrector1/1
  Ig_dq0*/1 -> vpcc_abc4/1, Demux/1
  Mux/1 -> vm/1

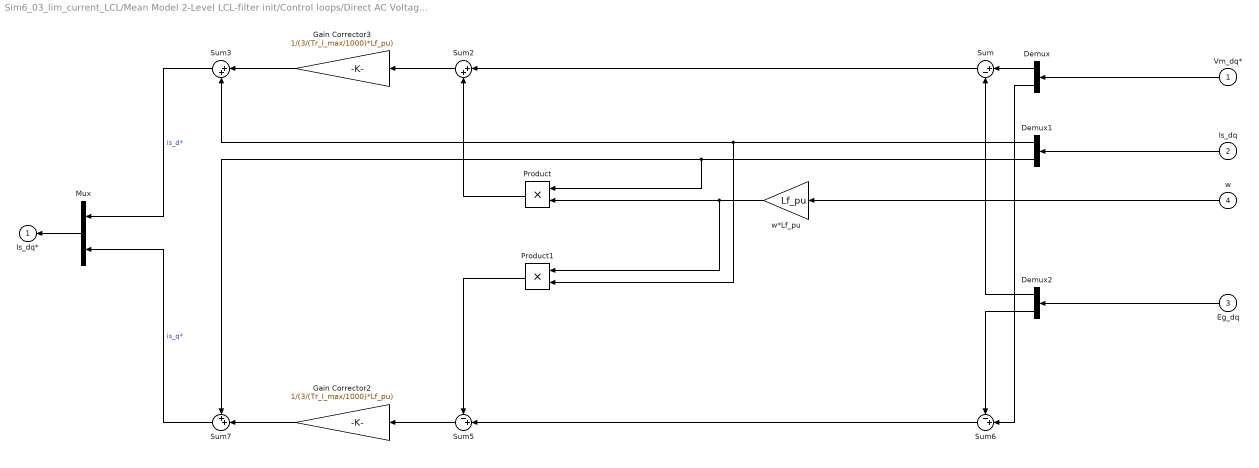
== system Sim6_03_lim_current_LCL/Mean Model 2-Level LCL-filter init/Control loops/Direct AC Voltage control/Current Limitation/Inverse Current control ==
  Vm_dq* : Inport
  Is_dq : Inport  Port=2
  Eg_dq : Inport  Port=3
  w : Inport  Port=4
  Demux : Demux  Outputs=2
  Demux1 : Demux  Outputs=2
  Demux2 : Demux  Outputs=2
  Gain Corrector2 : Gain  Gain=1/(3/(Tr_I_max/1000)*Lf_pu)
  Gain Corrector3 : Gain  Gain=1/(3/(Tr_I_max/1000)*Lf_pu)
  Mux : Mux  Inputs=2
  Product : Product  RndMeth=Zero
  Product1 : Product  RndMeth=Zero
  Sum : Sum  Inputs=|+-
  Sum2 : Sum  Inputs=|++
  Sum3 : Sum  Inputs=|++
  Sum5 : Sum  Inputs=-+|
  Sum6 : Sum  Inputs=-+|
  Sum7 : Sum  Inputs=++|
  w*Lf_pu : Gain  Gain=Lf_pu
  Is_dq* : Outport  InitialOutput=0  VectorParamsAs1DForOutWhenUnconnected=off
  wires:
  Eg_dq/1 -> Demux2/1
  Is_dq/1 -> Demux1/1
  Vm_dq*/1 -> Demux/1
  Demux/1 -> Sum/1
  Demux1/1 -> Sum3/2, Product1/2
  Sum/1 -> Sum2/1
  w*Lf_pu/1 -> Product1/1, Product/2
  Product/1 -> Sum2/2
  Sum2/1 -> Gain Corrector3/1
  Mux/1 -> Is_dq*/1
  Demux/2 -> Sum6/2
  Sum6/1 -> Sum5/2
  Sum5/1 -> Gain Corrector2/1
  Sum3/1 -> Mux/1  "is_d*"
  Sum7/1 -> Mux/2  "is_q*"
  w/1 -> w*Lf_pu/1
  Demux1/2 -> Sum7/1, Product/1
  Gain Corrector3/1 -> Sum3/1
  Demux2/1 -> Sum/2
  Demux2/2 -> Sum6/1
  Product1/1 -> Sum5/1
  Gain Corrector2/1 -> Sum7/2
